simulink model "Resonant"  (R2025a)
settings: Solver=VariableStepAuto  StartTime=0.0  StopTime=1  FixedStep=0.0001  RelTol=1e-3
undefined symbols (not defined in the file or in its folder): Angle, D1, Delta, Magnitude
libraries: spsCurrentMeasurementLib x16, spsThreePhasePISectionLineLib x10, spsThreePhaseTransformerTwoWindingsLib x7, spsThreePhaseSeriesRLCLoadLib x6, spsGroundLib x3, spsVoltageMeasurementLib x3, spsSeriesRLCBranchLib x1, spsThreePhaseVIMeasurementLib x1, spsThreePhaseFaultLib x1, spsThreePhaseSourceLib x1, spspowerguiLib x1
settings Model: SimulationMode=accelerator  Creator=ChengW  LastModifiedBy=19092
settings DataIOCC: ReturnWorkspaceOutputs=off
settings DebuggingCC: UnconnectedInputMsg=warning  UnconnectedOutputMsg=warning  UnconnectedLineMsg=warning  ArithmeticOperatorsInVariantConditions=warning
settings ModelReferenceCC: EnableRefExpFcnMdlSchedulingChecks=on
settings SFSimCC: SimUseLocalCustomCode=off  CustomCodeUndefinedFunction=UseInterfaceOnly
settings RTWCC: RTWUseLocalCustomCode=off  GPUComputeCapability=3.5

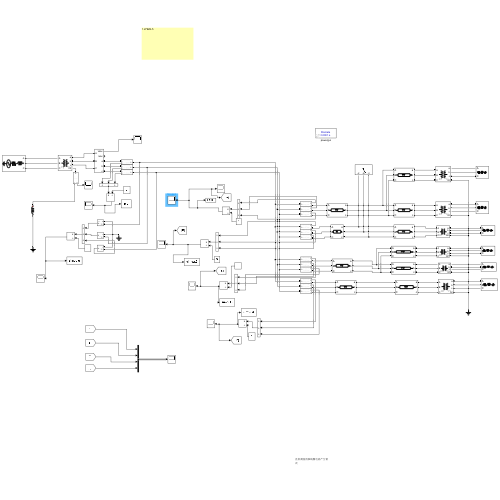
[thumbnail: Simulink's stored preview of the top-level diagram]
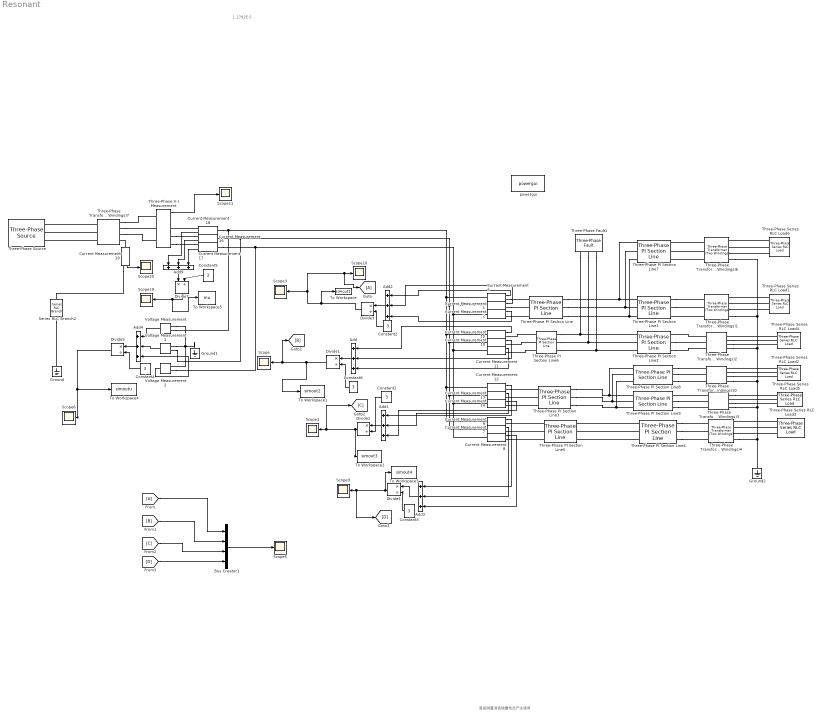
== system Resonant ==
  note: 直接测量消弧线圈电流产生错误
  note: 1.2792E-5
  Add{,1..4,9} (6 alike) : Sum  Inputs=+++
  Bus Creator1 : BusCreator  Inputs=4
  Constant{1..6} (6 alike) : Constant  Value=3
  Current Measurement{1..2,6..19} (16 alike) : spsCurrentMeasurementLib/Current Measurement  PhasorSimulation=off  OutputType=Magnitude-Angle  PSBequivalent=0
  Divide{1..5,7} (6 alike) : Product  Inputs=*/
  From : From
  Goto : Goto
  Ground : spsGroundLib/Ground  LConnTagsString=a
  Ground1 : spsGroundLib/Ground  LConnTagsString=a
  Ground2 : spsGroundLib/Ground  LConnTagsString=a
  Scope{,1,3,5..6,9..11,19..20} (10 alike) : Scope
      Scope settings: ActiveDisplayYMinimum=-8.27444756803148  ActiveDisplayYMaximum=-8.2744474560900283  DataLoggingVariableName=lingxudainliu2
      Scope1 settings: ActiveDisplayYMinimum=-18.143333397936757  ActiveDisplayYMaximum=16.740927007400572  DataLoggingVariableName=lingxudaunliu3
      Scope10 settings: ActiveDisplayYMinimum=-4.4087170491126386  ActiveDisplayYMaximum=3.5778101221384597  DataLoggingVariableName=ZAOlingxudianliu1
      Scope11 settings: ActiveDisplayYMinimum=-24021.63429298536  ActiveDisplayYMaximum=23391.378266070362
      Scope19 settings: ActiveDisplayYMinimum=-187.45232210313372  ActiveDisplayYMaximum=129.96322399315224  DataLoggingVariableName=ScopeData5
      Scope20 settings: ActiveDisplayYMinimum=-157.9397419355667  ActiveDisplayYMaximum=71.347391221722063
      Scope3 settings: ActiveDisplayYMinimum=-422.85139097357631  ActiveDisplayYMaximum=297.438439663776  DataLoggingVariableName=lingxudainliu1
      Scope5 settings: ActiveDisplayYMinimum=-55.84943  ActiveDisplayYMaximum=52.05941
      Scope6 settings: ActiveDisplayYMinimum=-11360.33274  ActiveDisplayYMaximum=9549.66393  DataLoggingVariableName=ScopeData3
      Scope9 settings: ActiveDisplayYMinimum=-8.97636  ActiveDisplayYMaximum=8.40917  DataLoggingVariableName=lingxudianliu4
  Series RLC Branch2 : spsSeriesRLCBranchLib/Series RLC Branch  LConnTagsString=__new0  RConnTagsString=__new0  BranchType=L  Resistance=100  Inductance=0.4452  SetiL0=off  InitialCurrent=0  Capacitance=1e-6  Setx0=off  InitialVoltage=0  Measurements=None
  Three-Phase PI Section Line : spsThreePhasePISectionLineLib/Three-Phase PI Section Line  LConnTagsString=a|b|c  RConnTagsString=A|B|C  Length=3  Frequency=50  Resistances=[0.27 2.7 ]  Inductances="[0.255e-3  1.109e-3]"  Capacitances=[0.376e-6 0.276e-6]
  Three-Phase PI Section Line1 : spsThreePhasePISectionLineLib/Three-Phase PI Section Line  LConnTagsString=a|b|c  RConnTagsString=A|B|C  Length=15  Frequency=50  Resistances=[0.17 0.32 ]  Inductances="[1.017e-3  3.56e-3]"  Capacitances=[0.115e-6 0.006e-6]
  Three-Phase PI Section Line2 : spsThreePhasePISectionLineLib/Three-Phase PI Section Line  LConnTagsString=a|b|c  RConnTagsString=A|B|C  Length=6  Frequency=50  Resistances=[0.27 2.7 ]  Inductances="[0.255e-3  1.109e-3]"  Capacitances=[0.376e-6 0.276e-6]
  Three-Phase PI Section Line3 : spsThreePhasePISectionLineLib/Three-Phase PI Section Line  LConnTagsString=a|b|c  RConnTagsString=A|B|C  Length=9  Frequency=50  Resistances=[0.27 2.7 ]  Inductances="[0.255e-3  1.109e-3]"  Capacitances=[0.376e-6 0.276e-6]
  Three-Phase PI Section Line4 : spsThreePhasePISectionLineLib/Three-Phase PI Section Line  LConnTagsString=a|b|c  RConnTagsString=A|B|C  Length=6  Frequency=50  Resistances=[0.17 0.32 ]  Inductances="[ 1.017e-3  3.56e-3]"  Capacitances=[0.115e-6 0.006e-6]
  Three-Phase PI Section Line5 : spsThreePhasePISectionLineLib/Three-Phase PI Section Line  LConnTagsString=a|b|c  RConnTagsString=A|B|C  Length=6  Frequency=50  Resistances=[0.27 2.7 ]  Inductances="[0.255e-3  1.109e-3]"  Capacitances=[0.376e-6 0.276e-6]
  Three-Phase PI Section Line6 : spsThreePhasePISectionLineLib/Three-Phase PI Section Line  LConnTagsString=a|b|c  RConnTagsString=A|B|C  Length=12  Frequency=50  Resistances=[0.17 0.32 ]  Inductances="[ 1.017e-3  3.56e-3]"  Capacitances=[0.115e-6 0.006e-6]
  Three-Phase PI Section Line7 : spsThreePhasePISectionLineLib/Three-Phase PI Section Line  LConnTagsString=a|b|c  RConnTagsString=A|B|C  Length=20  Frequency=50  Resistances=[0.17 0.32 ]  Inductances="[ 1.017e-3  3.56e-3]"  Capacitances=[0.115e-6 0.006e-6]
  Three-Phase PI Section Line8 : spsThreePhasePISectionLineLib/Three-Phase PI Section Line  LConnTagsString=a|b|c  RConnTagsString=A|B|C  Length=9  Frequency=50  Resistances=[0.17 0.32 ]  Inductances="[ 1.017e-3  3.56e-3]"  Capacitances=[0.115e-6 0.006e-6]
  Three-Phase PI Section Line9 : spsThreePhasePISectionLineLib/Three-Phase PI Section Line  LConnTagsString=a|b|c  RConnTagsString=A|B|C  Length=6  Frequency=50  Resistances=[0.17 0.32 ]  Inductances="[ 1.017e-3  3.56e-3]"  Capacitances=[0.115e-6 0.006e-6]
  Three-Phase Series RLC Load{1..6} (6 alike) : spsThreePhaseSeriesRLCLoadLib/Three-Phase Series RLC Load  LConnTagsString=A|B|C  Configuration=Delta  NominalVoltage=380  Vabc=[1e3 1e3 1e3]  Vabcp=[1e3 1e3 1e3]  NominalFrequency=50  UnbalancedPower=off  ActivePower=0.8e5  InductivePower=0.5e5  CapacitivePower=0.2e5  Pabc=[10e3 9e3 11e3]  QLabc=[100 90 110]  QCabc=[100 90 110]  Pabcp=[10e3 9e3 11e3]  QLabcp=[100 90 110]  QCabcp=[100 90 110]  Measurements=None  LoadType=constant Z
  Three-Phase Transformer (Two Windings){1..4,6,10} (6 alike) : spsThreePhaseTransformerTwoWindingsLib/Three-Phase Transformer (Two Windings)  Winding1Connection=Delta (D1)  Winding2Connection=Yn  CoreType=Three single-phase transformers  SetSaturation=off  Hysteresis=off  DataFile='hysteresis'  SetInitialFlux=off  Measurements=None  UNITS=SI  NominalPower=[5e6 , 50 ]  Winding1=[10e3 27.011 3.4392]  Winding2=[400 0.005 0.00063662]  Rm=6.7528e+06  Lm=21495  L0=0.5  Saturation=[0 0;0.10664 2292.3;44.435 2903.6]  InitialFluxes=[1528.2 -1528.2 1337.2]  BreakLoop=off  DiscreteSolver=Trapezoidal iterative  DataType=on  TransfoNumber=1
  Three-Phase Transformer (Two Windings)7 : spsThreePhaseTransformerTwoWindingsLib/Three-Phase Transformer (Two Windings)  Winding1Connection=Yg  Winding2Connection=Yn  CoreType=Three single-phase transformers  SetSaturation=off  Hysteresis=off  DataFile='hysteresis'  SetInitialFlux=off  Measurements=None  UNITS=SI  NominalPower=[ 30e6 , 50 ]  Winding1=[1.1e+05 0.242 0.030812]  Winding2=[11000 0.002 0.00025465]  Rm=60500  Lm=192.58  L0=0.5  Saturation=[0 0;1.7814 343.07;742.27 434.55]  InitialFluxes=[228.71 -228.71 200.12]  BreakLoop=off  DiscreteSolver=Trapezoidal iterative  DataType=on  TransfoNumber=1
  Three-Phase V-I Measurement : spsThreePhaseVIMeasurementLib/Three-Phase V-I Measurement  VoltageMeasurement=phase-to-ground  SetLabelV=off  LabelV=Vabc  Vpu=off  VpuLL=off  CurrentMeasurement=yes  SetLabelI=off  LabelI=Iabc  Ipu=off  Pbase=100e6  Vbase=500e3  OutputType=Complex  PhasorSimulation=off  PSBequivalent=0
  Three-Phase Fault1 : spsThreePhaseFaultLib/Three-Phase Fault  InitialStates=0  FaultA=on  FaultB=off  FaultC=off  GroundFault=on  SwitchTimes=0.135  External=off  SwitchStatus=NaN  FaultResistance=100  GroundResistance=0.000000001  SnubberResistance=1e6  SnubberCapacitance=inf  Measurements=None
  Three-Phase Source : spsThreePhaseSourceLib/Three-Phase Source  InternalConnection=Yg  VoltagePhases=off  Voltage=110e3  PhaseAngle=0  Voltage_phases=[25e3 25e3 25e3]/sqrt(3)  PhaseAngles_phases=[0 -120 +120]  Frequency=50  NonIdealSource=on  SpecifyImpedance=off  Resistance=0.8  Inductance=16.58e-3  ShortCircuitLevel=100e6  BaseVoltage=25e3  XRratio=7  BusType=swing  Pref=10e3  Qref=0  Prefabc=[10e3, 10e3, 10e3]  Qrefabc=[0, 0, 0]  Qmin=-inf  Qmax=inf
  To Workspace : ToWorkspace  VariableName=simout1  SaveFormat=Structure With Time  SampleTime=-1
  To Workspace1 : ToWorkspace  VariableName=simout2  SaveFormat=Structure With Time  SampleTime=-1
  To Workspace2 : ToWorkspace  VariableName=simout3  SaveFormat=Structure With Time  SampleTime=-1
  To Workspace3 : ToWorkspace  VariableName=simout4  SaveFormat=Structure With Time  SampleTime=-1
  To Workspace4 : ToWorkspace  VariableName=simoutu  SaveFormat=Structure With Time  SampleTime=-1
  To Workspace5 : ToWorkspace  VariableName=mu  SaveFormat=Structure With Time  SampleTime=-1
  Voltage Measurement : spsVoltageMeasurementLib/Voltage Measurement  PhasorSimulation=off  OutputType=Complex  PSBequivalent=0
  Voltage Measurement1 : spsVoltageMeasurementLib/Voltage Measurement  PhasorSimulation=off  OutputType=Complex  PSBequivalent=0
  Voltage Measurement2 : spsVoltageMeasurementLib/Voltage Measurement  PhasorSimulation=off  OutputType=Complex  PSBequivalent=0
  powergui : spspowerguiLib/powergui  Priority=1  SimulationMode=Discrete  SampleTime=0.0001  frequency=60  Iterations=50  frequencyindice=0  Pbase=100e6  ErrMax=1e-4  UnitsV=kV  UnitsW=MW  buscounter=0  FunctionMessages=off  echomessages=off  EnableUseOfTLC=off  CurrentSourceSwitches=off  DisableSnubberDevices=off  DisableRonSwitches=off  DisableVfSwitches=off  DisplayEquations=off  AutomaticDiscreteSolvers=off  SolverType=Tustin/Backward Euler (TBE)  Interpol=off  ExternalGateDelay=off  methode=off  Ts=100  x0status=blocks  SPID=off  SwTol=0  HookPort=off  NonlinearTolerance=1e-4  nMaxIteration=100  ContinueOnMaxIteration=off  RestoreLinks=warning  ResistiveCurrentMeasurement=off  Frange=[0:2:500]  Ylog=off  Xlog=off  ShowGrid=on  save=off  variable=ZData  structure=lingxudainliu1  ZoomFFT=off  StartTime=0.135  cycles=10  DisplayStyle=1  fundamental=50  FreqAxis=off  MaxFrequency=5000  frequencyindicesteady=1  RmsSteady=1  display=off
  wires:
  Add/1 -> Divide1/1
  Add1/1 -> Divide2/1
  Constant1/1 -> Divide2/2
  Add2/1 -> Divide3/1
  Add3/1 -> Divide4/1
  Constant3/1 -> Divide4/2
  [C] -> Bus Creator1/3
  [D] -> Bus Creator1/4
  Bus Creator1/1 -> Scope5/1
  [B] -> Bus Creator1/2
  Voltage Measurement/1 -> Add4/1
  Constant4/1 -> Divide5/2
  Add4/1 -> Divide5/1
  Voltage Measurement1/1 -> Add4/2
  Voltage Measurement2/1 -> Add4/3
  From/1 -> Bus Creator1/1
  Three-Phase V-I Measurement/1 -> Scope11/1
  Divide7/1 -> To Workspace5/1, Scope19/1
  Current Measurement19/1 -> Scope20/1
  Current Measurement18/1 -> Add9/1
  Current Measurement16/1 -> Add9/2
  Current Measurement17/1 -> Add9/3
  Add9/1 -> Divide7/1
  Constant5/1 -> Divide7/2
  Current Measurement6/1 -> Add2/1
  Current Measurement1/1 -> Add2/2
  Current Measurement2/1 -> Add2/3
  Constant2/1 -> Divide3/2
  Current Measurement15/1 -> Add/1
  Current Measurement10/1 -> Add/2
  Current Measurement11/1 -> Add/3
  Constant6/1 -> Divide1/2
  Current Measurement12/1 -> Add1/1
  Current Measurement13/1 -> Add1/2
  Current Measurement14/1 -> Add1/3
  Current Measurement9/1 -> Add3/1
  Current Measurement7/1 -> Add3/2
  Current Measurement8/1 -> Add3/3
  Divide1/1 -> [B], Scope/1, To Workspace1/1
  Divide2/1 -> [C], Scope1/1, To Workspace2/1
  Divide4/1 -> [D], Scope9/1, To Workspace3/1
  Divide5/1 -> To Workspace4/1, Scope6/1
  Divide3/1 -> To Workspace/1, Scope3/1, Goto/1, Scope10/1
  connections:
  Current Measurement6/RConn1 -- Three-Phase PI Section Line/LConn1
  Current Measurement1/RConn1 -- Three-Phase PI Section Line/LConn2
  Current Measurement2/RConn1 -- Three-Phase PI Section Line/LConn3
  Current Measurement12/LConn1 -- Current Measurement9/LConn1 -- Voltage Measurement/LConn1 -- Current Measurement18/LConn1 -- Current Measurement6/LConn1 -- Current Measurement15/LConn1
  Three-Phase PI Section Line/RConn2 -- Three-Phase PI Section Line7/LConn2 -- Three-Phase PI Section Line1/LConn2
  Three-Phase PI Section Line/RConn3 -- Three-Phase PI Section Line7/LConn3 -- Three-Phase PI Section Line1/LConn3
  Three-Phase Transformer (Two Windings)7/LConn1 -- Three-Phase Source/RConn1
  Three-Phase Transformer (Two Windings)7/LConn2 -- Three-Phase Source/RConn2
  Three-Phase Transformer (Two Windings)7/LConn3 -- Three-Phase Source/RConn3
  Three-Phase Transformer (Two Windings)7/RConn1 -- Three-Phase V-I Measurement/LConn1
  Three-Phase Transformer (Two Windings)7/RConn2 -- Three-Phase V-I Measurement/LConn2
  Three-Phase Transformer (Two Windings)7/RConn3 -- Three-Phase V-I Measurement/LConn3
  Current Measurement12/RConn1 -- Three-Phase PI Section Line3/LConn1
  Current Measurement13/RConn1 -- Three-Phase PI Section Line3/LConn2
  Current Measurement14/RConn1 -- Three-Phase PI Section Line3/LConn3
  Voltage Measurement1/LConn2 -- Ground1/LConn1 -- Voltage Measurement/LConn2 -- Voltage Measurement2/LConn2
  Three-Phase Transformer (Two Windings)1/RConn4 -- Three-Phase Transformer (Two Windings)6/RConn4 -- Ground2/LConn1 -- Three-Phase Transformer (Two Windings)4/RConn4 -- Three-Phase Transformer (Two Windings)3/RConn4 -- Three-Phase Transformer (Two Windings)10/RConn4 -- Three-Phase Transformer (Two Windings)2/RConn4
  Current Measurement18/RConn1 -- Three-Phase V-I Measurement/RConn1
  Three-Phase V-I Measurement/RConn2 -- Current Measurement16/RConn1
  Three-Phase V-I Measurement/RConn3 -- Current Measurement17/RConn1
  Current Measurement19/LConn1 -- Three-Phase Transformer (Two Windings)7/RConn4
  Current Measurement8/LConn1 -- Current Measurement11/LConn1 -- Voltage Measurement2/LConn1 -- Current Measurement17/LConn1 -- Current Measurement2/LConn1 -- Current Measurement14/LConn1
  Three-Phase Transformer (Two Windings)1/LConn3 -- Three-Phase PI Section Line1/RConn3
  Three-Phase PI Section Line1/RConn2 -- Three-Phase Transformer (Two Windings)1/LConn2
  Current Measurement7/LConn1 -- Voltage Measurement1/LConn1 -- Current Measurement16/LConn1 -- Current Measurement1/LConn1 -- Current Measurement10/LConn1 -- Current Measurement13/LConn1
  Series RLC Branch2/RConn1 -- Ground/LConn1
  Three-Phase PI Section Line1/RConn1 -- Three-Phase Transformer (Two Windings)1/LConn1
  Three-Phase Transformer (Two Windings)6/LConn2 -- Three-Phase PI Section Line7/RConn2
  Three-Phase Transformer (Two Windings)6/LConn3 -- Three-Phase PI Section Line7/RConn3
  Three-Phase Transformer (Two Windings)6/LConn1 -- Three-Phase PI Section Line7/RConn1
  Three-Phase Transformer (Two Windings)3/LConn1 -- Three-Phase PI Section Line9/RConn1
  Three-Phase PI Section Line9/RConn2 -- Three-Phase Transformer (Two Windings)3/LConn2
  Three-Phase PI Section Line9/RConn3 -- Three-Phase Transformer (Two Windings)3/LConn3
  Three-Phase Series RLC Load2/LConn1 -- Three-Phase Transformer (Two Windings)10/RConn1
  Three-Phase Transformer (Two Windings)10/RConn2 -- Three-Phase Series RLC Load2/LConn2
  Three-Phase Transformer (Two Windings)10/RConn3 -- Three-Phase Series RLC Load2/LConn3
  Three-Phase Series RLC Load3/LConn1 -- Three-Phase Transformer (Two Windings)4/RConn1
  Three-Phase Series RLC Load3/LConn2 -- Three-Phase Transformer (Two Windings)4/RConn2
  Three-Phase Series RLC Load3/LConn3 -- Three-Phase Transformer (Two Windings)4/RConn3
  Three-Phase PI Section Line/RConn1 -- Three-Phase PI Section Line7/LConn1 -- Three-Phase PI Section Line1/LConn1
  Three-Phase Series RLC Load6/LConn1 -- Three-Phase Transformer (Two Windings)6/RConn1
  Three-Phase Series RLC Load6/LConn2 -- Three-Phase Transformer (Two Windings)6/RConn2
  Three-Phase Series RLC Load6/LConn3 -- Three-Phase Transformer (Two Windings)6/RConn3
  Three-Phase PI Section Line6/LConn1 -- Current Measurement15/RConn1
  Three-Phase PI Section Line6/LConn3 -- Current Measurement11/RConn1
  Three-Phase PI Section Line6/LConn2 -- Current Measurement10/RConn1
  Three-Phase Transformer (Two Windings)2/LConn1 -- Three-Phase PI Section Line2/RConn1
  Three-Phase PI Section Line2/RConn2 -- Three-Phase Transformer (Two Windings)2/LConn2
  Three-Phase PI Section Line2/RConn3 -- Three-Phase Transformer (Two Windings)2/LConn3
  Three-Phase PI Section Line4/LConn1 -- Three-Phase PI Section Line5/RConn1
  Three-Phase PI Section Line4/LConn2 -- Three-Phase PI Section Line5/RConn2
  Three-Phase PI Section Line4/LConn3 -- Three-Phase PI Section Line5/RConn3
  Three-Phase PI Section Line4/RConn1 -- Three-Phase Transformer (Two Windings)4/LConn1
  Three-Phase PI Section Line4/RConn2 -- Three-Phase Transformer (Two Windings)4/LConn2
  Three-Phase PI Section Line4/RConn3 -- Three-Phase Transformer (Two Windings)4/LConn3
  Three-Phase PI Section Line5/LConn1 -- Current Measurement9/RConn1
  Three-Phase PI Section Line5/LConn2 -- Current Measurement7/RConn1
  Current Measurement8/RConn1 -- Three-Phase PI Section Line5/LConn3
  Three-Phase PI Section Line6/RConn1 -- Three-Phase Fault1/LConn1 -- Three-Phase PI Section Line2/LConn1
  Three-Phase PI Section Line6/RConn2 -- Three-Phase Fault1/LConn2 -- Three-Phase PI Section Line2/LConn2
  Three-Phase PI Section Line6/RConn3 -- Three-Phase Fault1/LConn3 -- Three-Phase PI Section Line2/LConn3
  Three-Phase Series RLC Load1/LConn1 -- Three-Phase Transformer (Two Windings)1/RConn1
  Three-Phase Series RLC Load1/LConn2 -- Three-Phase Transformer (Two Windings)1/RConn2
  Three-Phase Series RLC Load1/LConn3 -- Three-Phase Transformer (Two Windings)1/RConn3
  Three-Phase Series RLC Load4/LConn1 -- Three-Phase Transformer (Two Windings)2/RConn1
  Three-Phase Transformer (Two Windings)2/RConn2 -- Three-Phase Series RLC Load4/LConn2
  Three-Phase Transformer (Two Windings)2/RConn3 -- Three-Phase Series RLC Load4/LConn3
  Three-Phase Transformer (Two Windings)3/RConn1 -- Three-Phase Series RLC Load5/LConn1
  Three-Phase Series RLC Load5/LConn2 -- Three-Phase Transformer (Two Windings)3/RConn2
  Three-Phase Transformer (Two Windings)3/RConn3 -- Three-Phase Series RLC Load5/LConn3
  Three-Phase PI Section Line8/RConn1 -- Three-Phase Transformer (Two Windings)10/LConn1
  Three-Phase PI Section Line8/RConn2 -- Three-Phase Transformer (Two Windings)10/LConn2
  Three-Phase PI Section Line8/RConn3 -- Three-Phase Transformer (Two Windings)10/LConn3
  Three-Phase PI Section Line3/RConn1 -- Three-Phase PI Section Line8/LConn1 -- Three-Phase PI Section Line9/LConn1
  Three-Phase PI Section Line3/RConn2 -- Three-Phase PI Section Line8/LConn2 -- Three-Phase PI Section Line9/LConn2
  Three-Phase PI Section Line3/RConn3 -- Three-Phase PI Section Line8/LConn3 -- Three-Phase PI Section Line9/LConn3
  Current Measurement19/RConn1 -- Series RLC Branch2/LConn1
